simulink model "px4_multirotor_sim"  (R2019a)
settings: Solver=FixedStepAuto  StartTime=0.0  StopTime=sim_time  FixedStep=1/sim_freq  RelTol=1e-3
values from neighbouring files (symbols this model uses):
  C_D = [0.064; 0.067; 0.089].*0    [model_parameters.m]
  d = 0.49    [model_parameters.m]
  m = 4.5    [model_parameters.m]
  pos_e_step = [2;3;-4]    [setup_sim.m]
  r_D = 0.0237    [model_parameters.m]
  tau_T = 0.07    [model_parameters.m]
  virtual_controls_mat = [1 1 1 1; -1/sqrt(2) 1/sqrt(2) 1/sqrt(2) -1/sqrt(2); 1/sqrt(2) -1/sqrt(2) 1/sqrt(2) -1/sqrt(2); 1 1 -1 -1]    [model_parameters.m]
  wind = [0; 0; 0]    [model_parameters.m]
  yaw_step = 0    [setup_sim.m]
undefined symbols (not defined in the file or in its folder): br_filt_denom, br_filt_num, DiscIntNeverNeededParam, eta_w, g, hover_perc, hover_T, K_dp, K_ep, K_np, K_pd, K_phi, K_pi, K_pp, K_psi, K_qd, K_qi, K_qp, K_rd, K_ri, K_rp, K_theta, K_ud, K_ui, K_up, K_vd, K_vi, K_vp, K_wd, K_wi, K_wp, max_T, max_tilt, max_vel_xy, max_vel_z_down, max_vel_z_up, p_int_lim, p_max, q_int_lim, q_max, r_max, rho, thr_max, thr_min, vel_filt_denom, vel_filt_num
libraries: simulink x6, shared6dof x1, sharedtransform x1
settings Model: Creator=anton  LastModifiedBy=anton
settings DataIOCC: ReturnWorkspaceOutputs=off
settings DebuggingCC: ArithmeticOperatorsInVariantConditions=warning
settings ModelReferenceCC: ModelReferenceNumInstancesAllowed=Single

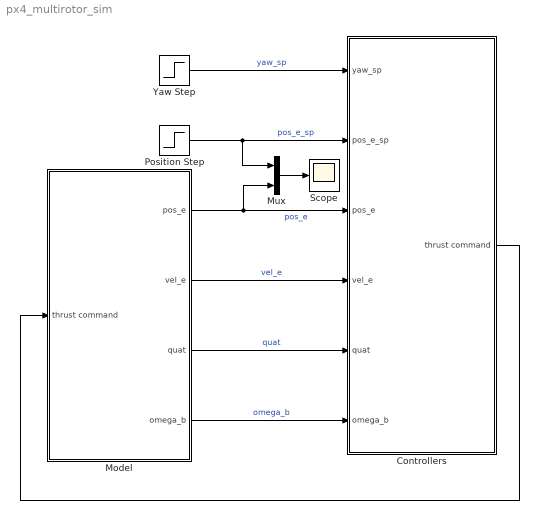
== system px4_multirotor_sim ==
  Controllers : Subsystem
  Model : Subsystem
  Mux : Mux  Inputs=2
  Position Step : Step  Before=[0;0;0]  After=pos_e_step  SampleTime=0
  Scope : Scope
  Yaw Step : Step  After=yaw_step  SampleTime=0
  wires:
  Controllers/1(thrust command) -> Model/1(thrust command)
  Model/1(pos_e) -> Mux/2, Controllers/3(pos_e)  "pos_e"
  Model/2(vel_e) -> Controllers/4(vel_e)  "vel_e"
  Model/3(quat) -> Controllers/5(quat)  "quat"
  Model/4(omega_b) -> Controllers/6(omega_b)  "omega_b"
  Position Step/1 -> Mux/1, Controllers/2(pos_e_sp)  "pos_e_sp"
  Yaw Step/1 -> Controllers/1(yaw_sp)  "yaw_sp"
  Mux/1 -> Scope/1

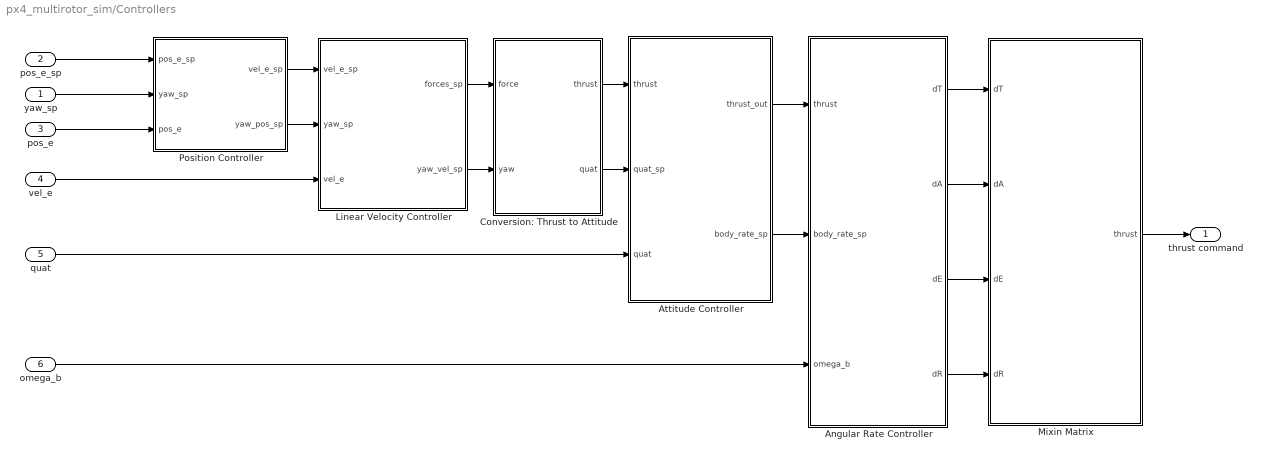
== system px4_multirotor_sim/Controllers ==
  yaw_sp : Inport
  pos_e_sp : Inport  Port=2
  pos_e : Inport  Port=3
  vel_e : Inport  Port=4
  quat : Inport  Port=5
  omega_b : Inport  Port=6
  Angular Rate Controller : Subsystem
  Attitude Controller : Subsystem
  Conversion: Thrust to Attitude : Subsystem
  Linear Velocity Controller : Subsystem
  Mixin Matrix : Subsystem
  Position Controller : Subsystem
  thrust command : Outport
  wires:
  Conversion: Thrust to Attitude/2(quat) -> Attitude Controller/2(quat_sp)
  Mixin Matrix/1(thrust) -> thrust command/1
  vel_e/1 -> Linear Velocity Controller/3(vel_e)
  Angular Rate Controller/3(dE) -> Mixin Matrix/3(dE)
  Attitude Controller/1(thrust_out) -> Angular Rate Controller/1(thrust)
  omega_b/1 -> Angular Rate Controller/3(omega_b)
  yaw_sp/1 -> Position Controller/2(yaw_sp)
  Linear Velocity Controller/2(yaw_vel_sp) -> Conversion: Thrust to Attitude/2(yaw)
  Angular Rate Controller/1(dT) -> Mixin Matrix/1(dT)
  pos_e_sp/1 -> Position Controller/1(pos_e_sp)
  Position Controller/1(vel_e_sp) -> Linear Velocity Controller/1(vel_e_sp)
  quat/1 -> Attitude Controller/3(quat)
  Angular Rate Controller/4(dR) -> Mixin Matrix/4(dR)
  Linear Velocity Controller/1(forces_sp) -> Conversion: Thrust to Attitude/1(force)
  pos_e/1 -> Position Controller/3(pos_e)
  Conversion: Thrust to Attitude/1(thrust) -> Attitude Controller/1(thrust)
  Position Controller/2(yaw_pos_sp) -> Linear Velocity Controller/2(yaw_sp)
  Angular Rate Controller/2(dA) -> Mixin Matrix/2(dA)
  Attitude Controller/2(body_rate_sp) -> Angular Rate Controller/2(body_rate_sp)

== system px4_multirotor_sim/Model ==
  thrust command : Inport
  6 DOF : Subsystem
  Forces and Moments : Subsystem
  Motor Model : Subsystem
  pos_e : Outport
  vel_e : Outport  Port=2
  quat : Outport  Port=3
  omega_b : Outport  Port=4
  wires:
  thrust command/1 -> Motor Model/1(thrust_cmd)
  Forces and Moments/2(moments) -> 6 DOF/2(moments)
  Forces and Moments/1(forces) -> 6 DOF/1(forces)
  6 DOF/1(pos_e) -> pos_e/1, Forces and Moments/1(pos_e)
  6 DOF/2(quat) -> quat/1, Forces and Moments/2(quat)
  6 DOF/3(vel_b) -> Forces and Moments/3(vel_b)
  6 DOF/4(omega_b) -> omega_b/1
  6 DOF/5(vel_e) -> vel_e/1
  Motor Model/1(force) -> Forces and Moments/4(Thrust Commands)

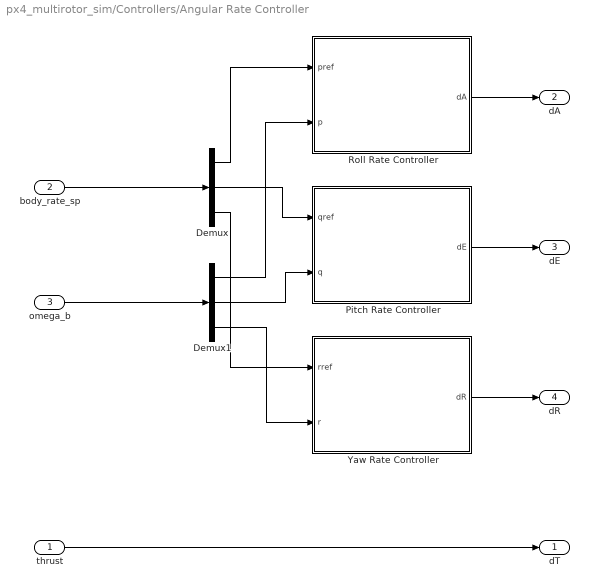
== system px4_multirotor_sim/Controllers/Angular Rate Controller ==
  thrust : Inport
  body_rate_sp : Inport  Port=2
  omega_b : Inport  Port=3
  Demux : Demux  Outputs=3
  Demux1 : Demux  Outputs=3
  Pitch Rate Controller : Subsystem
  Roll Rate Controller : Subsystem
  Yaw Rate Controller : Subsystem
  dT : Outport
  dA : Outport  Port=2
  dE : Outport  Port=3
  dR : Outport  Port=4
  wires:
  Demux1/3 -> Yaw Rate Controller/2(r)
  Demux/3 -> Yaw Rate Controller/1(rref)
  Demux1/1 -> Roll Rate Controller/2(p)
  thrust/1 -> dT/1
  Yaw Rate Controller/1(dR) -> dR/1
  Pitch Rate Controller/1(dE) -> dE/1
  Demux1/2 -> Pitch Rate Controller/2(q)
  Roll Rate Controller/1(dA) -> dA/1
  Demux/1 -> Roll Rate Controller/1(pref)
  Demux/2 -> Pitch Rate Controller/1(qref)
  omega_b/1 -> Demux1/1
  body_rate_sp/1 -> Demux/1

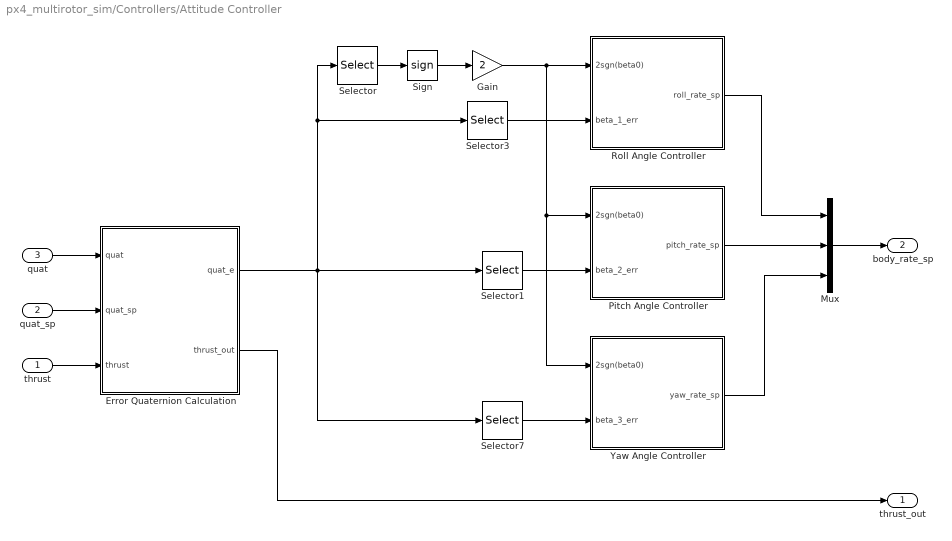
== system px4_multirotor_sim/Controllers/Attitude Controller ==
  thrust : Inport  PortDimensions=1
  quat_sp : Inport  Port=2  PortDimensions=4
  quat : Inport  Port=3  PortDimensions=4
  Error Quaternion Calculation : MATLAB Function  TreatAsAtomicUnit=on
  Gain : Gain  Gain=2
  Mux : Mux  Inputs=3
  Pitch Angle Controller : Subsystem
  Roll Angle Controller : Subsystem
  Selector : Selector  InputPortWidth=4  IndexOptions=Index vector (dialog)  Indices=1  OutputSizes=1
  Selector1 : Selector  InputPortWidth=4  IndexOptions=Index vector (dialog)  Indices=3  OutputSizes=1
  Selector3 : Selector  InputPortWidth=4  IndexOptions=Index vector (dialog)  Indices=2  OutputSizes=1
  Selector7 : Selector  InputPortWidth=4  IndexOptions=Index vector (dialog)  Indices=4  OutputSizes=1
  Sign : Signum
  Yaw Angle Controller : Subsystem
  thrust_out : Outport
  body_rate_sp : Outport  Port=2
  wires:
  Pitch Angle Controller/1(pitch_rate_sp) -> Mux/2
  Selector7/1 -> Yaw Angle Controller/2(beta_3_err)
  Mux/1 -> body_rate_sp/1
  quat/1 -> Error Quaternion Calculation/1(quat)
  quat_sp/1 -> Error Quaternion Calculation/2(quat_sp)
  Error Quaternion Calculation/1(quat_e) -> Selector7/1, Selector/1, Selector3/1, Selector1/1
  Selector/1 -> Sign/1
  Yaw Angle Controller/1(yaw_rate_sp) -> Mux/3
  Roll Angle Controller/1(roll_rate_sp) -> Mux/1
  Selector3/1 -> Roll Angle Controller/2(beta_1_err)
  Gain/1 -> Yaw Angle Controller/1(2sgn(beta0)), Pitch Angle Controller/1(2sgn(beta0)), Roll Angle Controller/1(2sgn(beta0))
  thrust/1 -> Error Quaternion Calculation/3(thrust)
  Sign/1 -> Gain/1
  Error Quaternion Calculation/2(thrust_out) -> thrust_out/1
  Selector1/1 -> Pitch Angle Controller/2(beta_2_err)

== system px4_multirotor_sim/Controllers/Conversion: Thrust to Attitude ==
  force : Inport
  yaw : Inport  Port=2
  thrust2att : MATLAB Function  TreatAsAtomicUnit=on
  thrust : Outport
  quat : Outport  Port=2
  wires:
  yaw/1 -> thrust2att/2(yaw)
  force/1 -> thrust2att/1(force)
  thrust2att/2(thrust) -> thrust/1
  thrust2att/1(quat) -> quat/1

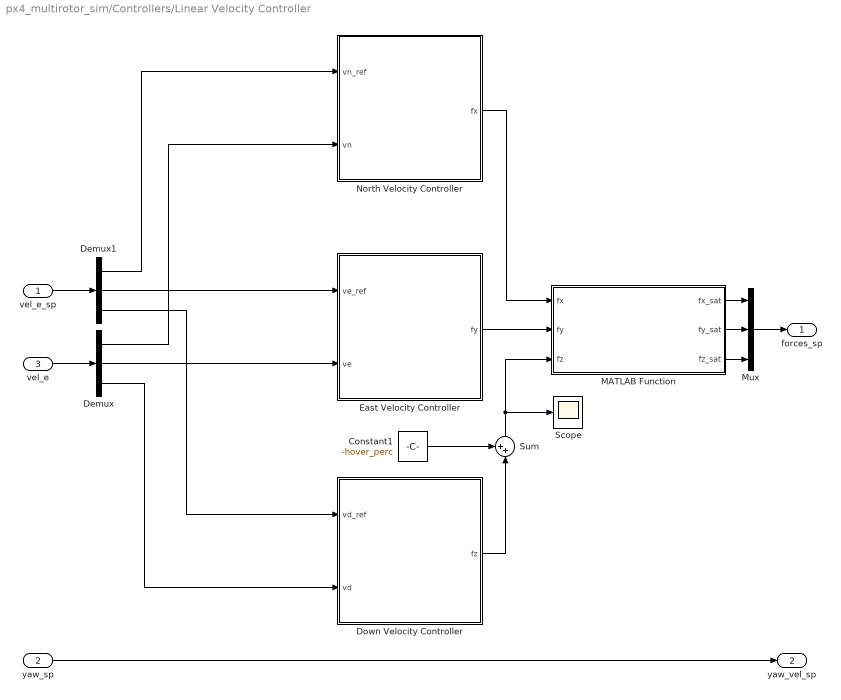
== system px4_multirotor_sim/Controllers/Linear Velocity Controller ==
  vel_e_sp : Inport
  yaw_sp : Inport  Port=2
  vel_e : Inport  Port=3
  Constant1 : Constant  Value=-hover_perc
  Demux : Demux  Outputs=3
  Demux1 : Demux  Outputs=3
  Down Velocity Controller : Subsystem
  East Velocity Controller : Subsystem
  MATLAB Function : MATLAB Function  TreatAsAtomicUnit=on
  Mux : Mux  Inputs=3
  North Velocity Controller : Subsystem
  Scope : Scope
  Sum : Sum  Inputs=++|
  forces_sp : Outport
  yaw_vel_sp : Outport  Port=2
  wires:
  Mux/1 -> forces_sp/1
  Demux/2 -> East Velocity Controller/2(ve)
  vel_e_sp/1 -> Demux1/1
  Down Velocity Controller/1(fz) -> Sum/2
  Demux1/1 -> North Velocity Controller/1(vn_ref)
  Constant1/1 -> Sum/1
  Demux/1 -> North Velocity Controller/2(vn)
  Demux/3 -> Down Velocity Controller/2(vd)
  vel_e/1 -> Demux/1
  MATLAB Function/1(fx_sat) -> Mux/1
  East Velocity Controller/1(fy) -> MATLAB Function/2(fy)
  North Velocity Controller/1(fx) -> MATLAB Function/1(fx)
  yaw_sp/1 -> yaw_vel_sp/1
  Demux1/3 -> Down Velocity Controller/1(vd_ref)
  Demux1/2 -> East Velocity Controller/1(ve_ref)
  MATLAB Function/3(fz_sat) -> Mux/3
  Sum/1 -> Scope/1, MATLAB Function/3(fz)
  MATLAB Function/2(fy_sat) -> Mux/2

== system px4_multirotor_sim/Controllers/Mixin Matrix ==
  dT : Inport
  dA : Inport  Port=2
  dE : Inport  Port=3
  dR : Inport  Port=4
  MATLAB Function : MATLAB Function  TreatAsAtomicUnit=on
  Precision Conversion : Subsystem
  Saturation : Saturate  UpperLimit=1  LowerLimit=0
  thrust : Outport
  wires:
  MATLAB Function/1(thrust) -> Saturation/1
  dT/1 -> MATLAB Function/1(dT)
  Saturation/1 -> Precision Conversion/1(analog_cmd)
  dE/1 -> MATLAB Function/3(dE)
  dA/1 -> MATLAB Function/2(dA)
  dR/1 -> MATLAB Function/4(dR)
  Precision Conversion/1(discrete_cmd) -> thrust/1

== system px4_multirotor_sim/Controllers/Position Controller ==
  pos_e_sp : Inport
  yaw_sp : Inport  Port=2
  pos_e : Inport  Port=3
  Demux : Demux  Outputs=3
  Demux1 : Demux  Outputs=3
  Down Position Controller : Subsystem
  East Position Controller : Subsystem
  Mux : Mux  Inputs=3
  North Position Controller : Subsystem
  vel_e_sp : Outport
  yaw_pos_sp : Outport  Port=2
  wires:
  Demux/1 -> North Position Controller/1(n_ref)
  North Position Controller/1(vn) -> Mux/1
  pos_e_sp/1 -> Demux/1
  yaw_sp/1 -> yaw_pos_sp/1
  Demux1/1 -> North Position Controller/2(n)
  Demux/2 -> East Position Controller/1(e_ref)
  Down Position Controller/1(vd) -> Mux/3
  Demux1/2 -> East Position Controller/2(e)
  Demux/3 -> Down Position Controller/1(d_ref)
  Mux/1 -> vel_e_sp/1
  East Position Controller/1(ve) -> Mux/2
  Demux1/3 -> Down Position Controller/2(d)
  pos_e/1 -> Demux1/1

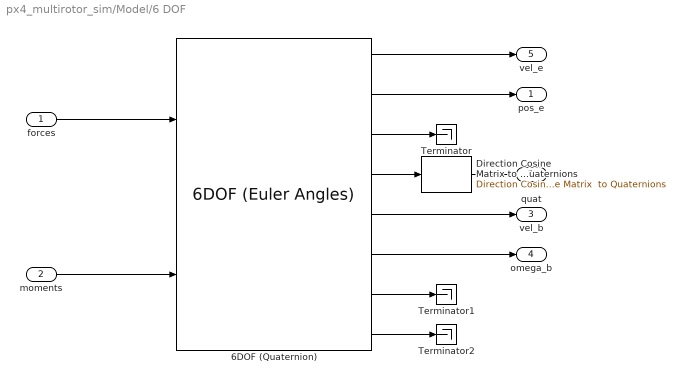
== system px4_multirotor_sim/Model/6 DOF ==
  forces : Inport
  moments : Inport  Port=2
  6DOF (Quaternion) : shared6dof/6DOF (Euler Angles)  units=Metric (MKS)  mtype=Fixed  rep=Quaternion  xme_0=[0 0 0]  Vm_0=[0 0 0]  eul_0=[0 0 0]  pm_0=[0 0 0]  mass_0=m  mass_e=0.5  mass_f=2.0  inertia=I  inertia_e=eye(3)  inertia_f=2*eye(3)  k_quat=2  vre_flag=on  abi_flag=off  aMode=0  xme_statename=''  Vm_statename=''  eul_statename=''  quat_statename=''  pm_statename=''  mass_statename=''
      settings: SourceProductBaseCode=AE
  Direction Cosine Matrix to Quaternions : sharedtransform/Direction Cosine Matrix  to Quaternions  aMode=0  action=None  tolerance=eps(2)
      settings: SourceProductName=Aerospace Blockset  SourceProductBaseCode=AE
  Terminator : Terminator
  Terminator1 : Terminator
  Terminator2 : Terminator
  pos_e : Outport
  quat : Outport  Port=2
  vel_b : Outport  Port=3
  omega_b : Outport  Port=4
  vel_e : Outport  Port=5
  wires:
  6DOF (Quaternion)/4 -> Direction Cosine Matrix to Quaternions/1
  6DOF (Quaternion)/1 -> vel_e/1
  Direction Cosine Matrix to Quaternions/1 -> quat/1
  forces/1 -> 6DOF (Quaternion)/1
  6DOF (Quaternion)/6 -> omega_b/1
  6DOF (Quaternion)/2 -> pos_e/1
  6DOF (Quaternion)/5 -> vel_b/1
  6DOF (Quaternion)/7 -> Terminator1/1
  6DOF (Quaternion)/3 -> Terminator/1
  moments/1 -> 6DOF (Quaternion)/2
  6DOF (Quaternion)/8 -> Terminator2/1

== system px4_multirotor_sim/Model/Forces and Moments ==
  pos_e : Inport
  quat : Inport  Port=2
  vel_b : Inport  Port=3
  Thrust Commands : Inport  Port=4
  Aerodynamic Model : Subsystem
  Gravity Model : Subsystem
  Sum : Sum  Inputs=|+++|
  Sum1 : Sum  Inputs=|+++|
  Thrust Model : Subsystem
  forces : Outport
  moments : Outport  Port=2
  wires:
  Thrust Model/2(moments) -> Sum1/2
  Gravity Model/2(moments) -> Sum1/3
  Gravity Model/1(forces) -> Sum/3
  Aerodynamic Model/2(moments) -> Sum1/1
  Aerodynamic Model/1(forces) -> Sum/1
  Thrust Model/1(forces) -> Sum/2
  Sum/1 -> forces/1
  Sum1/1 -> moments/1
  vel_b/1 -> Aerodynamic Model/1(vel_b)
  pos_e/1 -> Aerodynamic Model/2(pos_e)
  quat/1 -> Gravity Model/1(quat), Aerodynamic Model/3(quat)
  Thrust Commands/1 -> Thrust Model/1(Thrust Commands)

== system px4_multirotor_sim/Model/Motor Model ==
  thrust_cmd : Inport
  Linear Gain : Gain  Gain=max_T
  force : Outport
  wires:
  thrust_cmd/1 -> Linear Gain/1
  Linear Gain/1 -> force/1

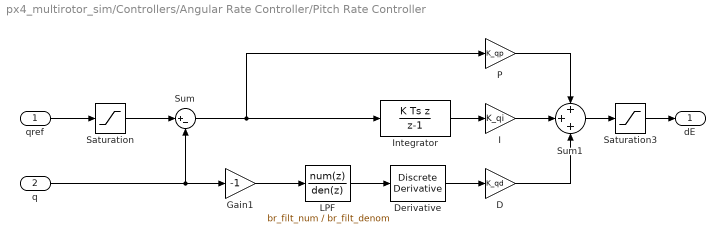
== system px4_multirotor_sim/Controllers/Angular Rate Controller/Pitch Rate Controller ==
  qref : Inport
  q : Inport  Port=2
  D : Gain  Gain=K_qd
  Derivative : simulink/Discrete/Discrete Derivative  gainval=1  ICPrevScaledInput=0.0  OutMin=[]  OutMax=[]  OutDataType=fixdt(1, 16)  OutScaling=2^-10  DoSatur=off
  Gain1 : Gain  Gain=-1
  I : Gain  Gain=K_qi
  Integrator : DiscreteIntegrator  IntegratorMethod=Integration: Backward Euler  gainval=1  SampleTime=-1  LimitOutput=on  UpperSaturationLimit=p_int_lim  LowerSaturationLimit=-p_int_lim  ICPrevOutput=DiscIntNeverNeededParam  ICPrevScaledInput=DiscIntNeverNeededParam
  LPF : DiscreteTransferFcn  Numerator=br_filt_num  Denominator=br_filt_denom
  P : Gain  Gain=K_qp
  Saturation : Saturate  UpperLimit=q_max  LowerLimit=-q_max
  Saturation3 : Saturate  UpperLimit=1  LowerLimit=-1
  Sum : Sum  Inputs=|+-
  Sum1 : Sum  Inputs=+++
  dE : Outport
  wires:
  Gain1/1 -> LPF/1
  P/1 -> Sum1/1
  Sum1/1 -> Saturation3/1
  Saturation/1 -> Sum/1
  I/1 -> Sum1/2
  Sum/1 -> Integrator/1, P/1
  Derivative/1 -> D/1
  D/1 -> Sum1/3
  qref/1 -> Saturation/1
  q/1 -> Gain1/1, Sum/2
  LPF/1 -> Derivative/1
  Integrator/1 -> I/1
  Saturation3/1 -> dE/1

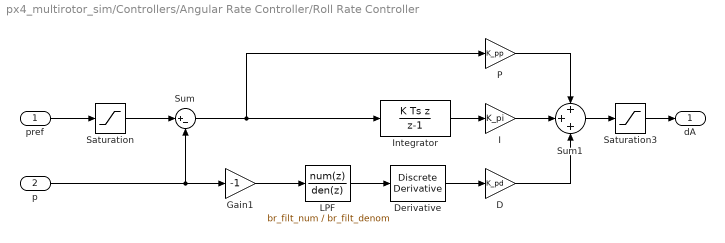
== system px4_multirotor_sim/Controllers/Angular Rate Controller/Roll Rate Controller ==
  pref : Inport
  p : Inport  Port=2
  D : Gain  Gain=K_pd
  Derivative : simulink/Discrete/Discrete Derivative  gainval=1  ICPrevScaledInput=0.0  OutMin=[]  OutMax=[]  OutDataType=fixdt(1, 16)  OutScaling=2^-10  DoSatur=off
  Gain1 : Gain  Gain=-1
  I : Gain  Gain=K_pi
  Integrator : DiscreteIntegrator  IntegratorMethod=Integration: Backward Euler  gainval=1  SampleTime=-1  LimitOutput=on  UpperSaturationLimit=p_int_lim  LowerSaturationLimit=-p_int_lim  ICPrevOutput=DiscIntNeverNeededParam  ICPrevScaledInput=DiscIntNeverNeededParam
  LPF : DiscreteTransferFcn  Numerator=br_filt_num  Denominator=br_filt_denom
  P : Gain  Gain=K_pp
  Saturation : Saturate  UpperLimit=p_max  LowerLimit=-p_max
  Saturation3 : Saturate  UpperLimit=1  LowerLimit=-1
  Sum : Sum  Inputs=|+-
  Sum1 : Sum  Inputs=+++
  dA : Outport
  wires:
  Gain1/1 -> LPF/1
  P/1 -> Sum1/1
  Sum1/1 -> Saturation3/1
  Saturation/1 -> Sum/1
  I/1 -> Sum1/2
  Sum/1 -> Integrator/1, P/1
  Derivative/1 -> D/1
  D/1 -> Sum1/3
  pref/1 -> Saturation/1
  p/1 -> Gain1/1, Sum/2
  LPF/1 -> Derivative/1
  Integrator/1 -> I/1
  Saturation3/1 -> dA/1

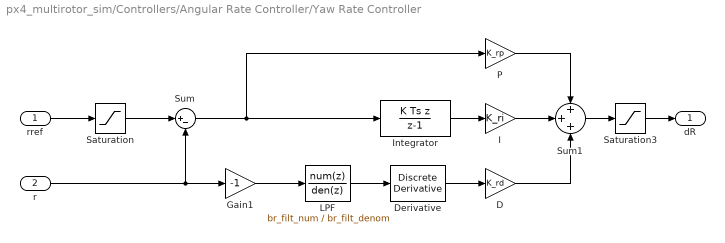
== system px4_multirotor_sim/Controllers/Angular Rate Controller/Yaw Rate Controller ==
  rref : Inport
  r : Inport  Port=2
  D : Gain  Gain=K_rd
  Derivative : simulink/Discrete/Discrete Derivative  gainval=1  ICPrevScaledInput=0.0  OutMin=[]  OutMax=[]  OutDataType=fixdt(1, 16)  OutScaling=2^-10  DoSatur=off
  Gain1 : Gain  Gain=-1
  I : Gain  Gain=K_ri
  Integrator : DiscreteIntegrator  IntegratorMethod=Integration: Backward Euler  gainval=1  SampleTime=-1  LimitOutput=on  UpperSaturationLimit=p_int_lim  LowerSaturationLimit=-p_int_lim  ICPrevOutput=DiscIntNeverNeededParam  ICPrevScaledInput=DiscIntNeverNeededParam
  LPF : DiscreteTransferFcn  Numerator=br_filt_num  Denominator=br_filt_denom
  P : Gain  Gain=K_rp
  Saturation : Saturate  UpperLimit=r_max  LowerLimit=-r_max
  Saturation3 : Saturate  UpperLimit=1  LowerLimit=-1
  Sum : Sum  Inputs=|+-
  Sum1 : Sum  Inputs=+++
  dR : Outport
  wires:
  Gain1/1 -> LPF/1
  P/1 -> Sum1/1
  Sum1/1 -> Saturation3/1
  Saturation/1 -> Sum/1
  I/1 -> Sum1/2
  Sum/1 -> Integrator/1, P/1
  Derivative/1 -> D/1
  D/1 -> Sum1/3
  rref/1 -> Saturation/1
  r/1 -> Gain1/1, Sum/2
  LPF/1 -> Derivative/1
  Integrator/1 -> I/1
  Saturation3/1 -> dR/1

== system px4_multirotor_sim/Controllers/Attitude Controller/Pitch Angle Controller ==
  2sgn(beta0) : Inport
  beta_2_err : Inport  Port=2
  Multiply : Product
  P : Gain  Gain=K_theta
  pitch_rate_sp : Outport
  wires:
  P/1 -> Multiply/1
  beta_2_err/1 -> P/1
  2sgn(beta0)/1 -> Multiply/2
  Multiply/1 -> pitch_rate_sp/1

== system px4_multirotor_sim/Controllers/Attitude Controller/Roll Angle Controller ==
  2sgn(beta0) : Inport
  beta_1_err : Inport  Port=2
  Multiply : Product
  P : Gain  Gain=K_phi
  roll_rate_sp : Outport
  wires:
  P/1 -> Multiply/1
  beta_1_err/1 -> P/1
  2sgn(beta0)/1 -> Multiply/2
  Multiply/1 -> roll_rate_sp/1

== system px4_multirotor_sim/Controllers/Attitude Controller/Yaw Angle Controller ==
  2sgn(beta0) : Inport
  beta_3_err : Inport  Port=2
  Multiply : Product
  P : Gain  Gain=K_psi
  yaw_rate_sp : Outport
  wires:
  P/1 -> Multiply/1
  beta_3_err/1 -> P/1
  2sgn(beta0)/1 -> Multiply/2
  Multiply/1 -> yaw_rate_sp/1

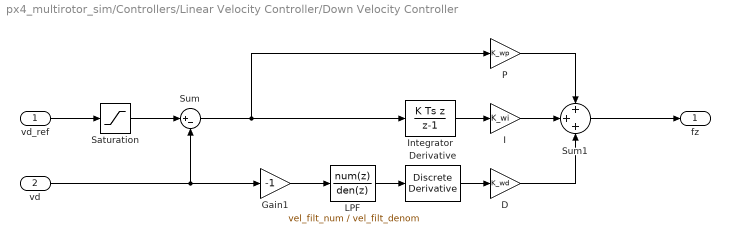
== system px4_multirotor_sim/Controllers/Linear Velocity Controller/Down Velocity Controller ==
  vd_ref : Inport
  vd : Inport  Port=2
  D : Gain  Gain=K_wd
  Derivative : simulink/Discrete/Discrete Derivative  gainval=1  ICPrevScaledInput=0.0  OutMin=[]  OutMax=[]  OutDataType=fixdt(1, 16)  OutScaling=2^-10  DoSatur=off
  Gain1 : Gain  Gain=-1
  I : Gain  Gain=K_wi
  Integrator : DiscreteIntegrator  IntegratorMethod=Integration: Backward Euler  gainval=1  SampleTime=-1  UpperSaturationLimit=q_int_lim  LowerSaturationLimit=-q_int_lim  ICPrevOutput=DiscIntNeverNeededParam  ICPrevScaledInput=DiscIntNeverNeededParam
  LPF : DiscreteTransferFcn  Numerator=vel_filt_num  Denominator=vel_filt_denom
  P : Gain  Gain=K_wp
  Saturation : Saturate  UpperLimit=max_vel_z_up  LowerLimit=max_vel_z_down
  Sum : Sum  Inputs=|+-
  Sum1 : Sum  Inputs=+++
  fz : Outport
  wires:
  vd_ref/1 -> Saturation/1
  P/1 -> Sum1/1
  Sum1/1 -> fz/1
  vd/1 -> Sum/2, Gain1/1
  Gain1/1 -> LPF/1
  LPF/1 -> Derivative/1
  D/1 -> Sum1/3
  Saturation/1 -> Sum/1
  I/1 -> Sum1/2
  Integrator/1 -> I/1
  Sum/1 -> Integrator/1, P/1
  Derivative/1 -> D/1

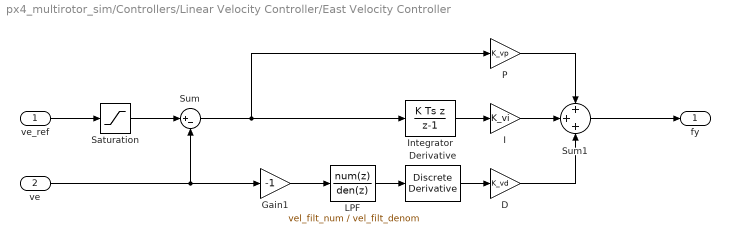
== system px4_multirotor_sim/Controllers/Linear Velocity Controller/East Velocity Controller ==
  ve_ref : Inport
  ve : Inport  Port=2
  D : Gain  Gain=K_vd
  Derivative : simulink/Discrete/Discrete Derivative  gainval=1  ICPrevScaledInput=0.0  OutMin=[]  OutMax=[]  OutDataType=fixdt(1, 16)  OutScaling=2^-10  DoSatur=off
  Gain1 : Gain  Gain=-1
  I : Gain  Gain=K_vi
  Integrator : DiscreteIntegrator  IntegratorMethod=Integration: Backward Euler  gainval=1  SampleTime=-1  UpperSaturationLimit=q_int_lim  LowerSaturationLimit=-q_int_lim  ICPrevOutput=DiscIntNeverNeededParam  ICPrevScaledInput=DiscIntNeverNeededParam
  LPF : DiscreteTransferFcn  Numerator=vel_filt_num  Denominator=vel_filt_denom
  P : Gain  Gain=K_vp
  Saturation : Saturate  UpperLimit=max_vel_xy  LowerLimit=-max_vel_xy
  Sum : Sum  Inputs=|+-
  Sum1 : Sum  Inputs=+++
  fy : Outport
  wires:
  ve_ref/1 -> Saturation/1
  P/1 -> Sum1/1
  Sum1/1 -> fy/1
  ve/1 -> Sum/2, Gain1/1
  Gain1/1 -> LPF/1
  LPF/1 -> Derivative/1
  D/1 -> Sum1/3
  Saturation/1 -> Sum/1
  I/1 -> Sum1/2
  Integrator/1 -> I/1
  Sum/1 -> Integrator/1, P/1
  Derivative/1 -> D/1

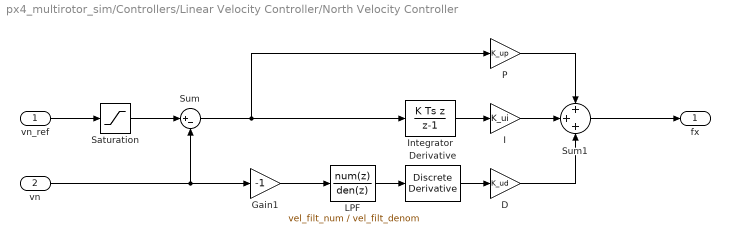
== system px4_multirotor_sim/Controllers/Linear Velocity Controller/North Velocity Controller ==
  vn_ref : Inport
  vn : Inport  Port=2
  D : Gain  Gain=K_ud
  Derivative : simulink/Discrete/Discrete Derivative  gainval=1  ICPrevScaledInput=0.0  OutMin=[]  OutMax=[]  OutDataType=fixdt(1, 16)  OutScaling=2^-10  DoSatur=off
  Gain1 : Gain  Gain=-1
  I : Gain  Gain=K_ui
  Integrator : DiscreteIntegrator  IntegratorMethod=Integration: Backward Euler  gainval=1  SampleTime=-1  UpperSaturationLimit=q_int_lim  LowerSaturationLimit=-q_int_lim  ICPrevOutput=DiscIntNeverNeededParam  ICPrevScaledInput=DiscIntNeverNeededParam
  LPF : DiscreteTransferFcn  Numerator=vel_filt_num  Denominator=vel_filt_denom
  P : Gain  Gain=K_up
  Saturation : Saturate  UpperLimit=max_vel_xy  LowerLimit=-max_vel_xy
  Sum : Sum  Inputs=|+-
  Sum1 : Sum  Inputs=+++
  fx : Outport
  wires:
  vn_ref/1 -> Saturation/1
  P/1 -> Sum1/1
  Sum1/1 -> fx/1
  vn/1 -> Sum/2, Gain1/1
  LPF/1 -> Derivative/1
  D/1 -> Sum1/3
  Saturation/1 -> Sum/1
  I/1 -> Sum1/2
  Integrator/1 -> I/1
  Sum/1 -> Integrator/1, P/1
  Derivative/1 -> D/1
  Gain1/1 -> LPF/1

== system px4_multirotor_sim/Controllers/Mixin Matrix/Precision Conversion ==
  analog_cmd : Inport
  Gain : Gain  Gain=10000
  Gain1 : Gain  Gain=1/10000
  Round : Rounding
  discrete_cmd : Outport
  wires:
  analog_cmd/1 -> Gain/1
  Gain/1 -> Round/1
  Round/1 -> Gain1/1
  Gain1/1 -> discrete_cmd/1

== system px4_multirotor_sim/Controllers/Position Controller/Down Position Controller ==
  d_ref : Inport
  d : Inport  Port=2
  P : Gain  Gain=K_dp
  Sum : Sum  Inputs=|+-
  vd : Outport
  wires:
  d/1 -> Sum/2
  d_ref/1 -> Sum/1
  Sum/1 -> P/1
  P/1 -> vd/1

== system px4_multirotor_sim/Controllers/Position Controller/East Position Controller ==
  e_ref : Inport
  e : Inport  Port=2
  P : Gain  Gain=K_ep
  Sum : Sum  Inputs=|+-
  ve : Outport
  wires:
  e/1 -> Sum/2
  e_ref/1 -> Sum/1
  Sum/1 -> P/1
  P/1 -> ve/1

== system px4_multirotor_sim/Controllers/Position Controller/North Position Controller ==
  n_ref : Inport
  n : Inport  Port=2
  P : Gain  Gain=K_np
  Sum : Sum  Inputs=|+-
  vn : Outport
  wires:
  n/1 -> Sum/2
  n_ref/1 -> Sum/1
  Sum/1 -> P/1
  P/1 -> vn/1

== system px4_multirotor_sim/Model/Forces and Moments/Aerodynamic Model ==
  vel_b : Inport
  pos_e : Inport  Port=2
  quat : Inport  Port=3
  Constant : Constant  Value=wind
  MATLAB Function : MATLAB Function  TreatAsAtomicUnit=on
  forces : Outport
  moments : Outport  Port=2
  wires:
  Constant/1 -> MATLAB Function/2(vw_i)
  MATLAB Function/2(moments) -> moments/1
  quat/1 -> MATLAB Function/4(quat)
  vel_b/1 -> MATLAB Function/1(v_b)
  pos_e/1 -> MATLAB Function/3(ned)
  MATLAB Function/1(forces) -> forces/1

== system px4_multirotor_sim/Model/Forces and Moments/Gravity Model ==
  quat : Inport
  MATLAB Function : MATLAB Function  TreatAsAtomicUnit=on
  forces : Outport
  moments : Outport  Port=2
  wires:
  MATLAB Function/2(moments) -> moments/1
  MATLAB Function/1(forces) -> forces/1
  quat/1 -> MATLAB Function/1(quat)

== system px4_multirotor_sim/Model/Forces and Moments/Thrust Model ==
  Thrust Commands : Inport
  Integrator : Integrator  InitialCondition=hover_T * ones(4,1)
  MATLAB Function : MATLAB Function  TreatAsAtomicUnit=on
  forces : Outport
  moments : Outport  Port=2
  wires:
  MATLAB Function/1(T_dot) -> Integrator/1
  Integrator/1 -> MATLAB Function/1(T)
  Thrust Commands/1 -> MATLAB Function/2(Tc)
  MATLAB Function/2(forces) -> forces/1
  MATLAB Function/3(moments) -> moments/1

== matlab function px4_multirotor_sim/Model/Forces and Moments/Aerodynamic Model/MATLAB Function ==
  data: v_b input size=3; vw_i input size=3; ned input size=3; quat input size=4; rho parameter size=1; forces output size=3; moments output size=3; C_D parameter size=3; eta_w parameter size=1
function [forces, moments] = aerodynamicModel(v_b, vw_i, ned, quat, rho, C_D, eta_w)
    coder.extrinsic("quatrotate");
    
    % Initialize
    vw_b = [0; 0; 0];
    
    vw_b = quatrotate(quat', vw_i')';
    vw_bm = (power(abs(ned(3))/10, eta_w)) .* vw_b;
    v_bw = -v_b + vw_bm;
    q = 0.5 * rho * v_bw.*abs(v_bw);
    
    forces = q.*C_D;
    moments = [0; 0; 0];
    
end

== matlab function px4_multirotor_sim/Model/Forces and Moments/Thrust Model/MATLAB Function ==
  data: T input size=4; T_dot output size=4; Tc input size=4; tau_T parameter size=1; forces output size=3; moments output size=3; d parameter size=1; r_D parameter size=1; virtual_controls_mat parameter size=[4,4]
function [T_dot, forces, moments]  = thrustModel(T, Tc, tau_T, d, r_D, virtual_controls_mat)

    virt_T = virtual_controls_mat * T;

    T_dot = (-T + Tc)/tau_T;
    forces = [0; 0; -virt_T(1)];
    moments = [d*virt_T(2); d*virt_T(3); r_D*virt_T(4)];
    
end

== matlab function px4_multirotor_sim/Model/Forces and Moments/Gravity Model/MATLAB Function ==
  data: quat input size=4; forces output size=3; moments output size=3; m parameter size=1; g parameter size=1
function [forces,moments] = gravitationalModel(quat, m, g)
    coder.extrinsic("quatrotate");

    % Initialize
    forces = [0; 0; 0];
    
    moments = [0 ; 0 ; 0];
    forces = quatrotate(quat', [0 ; 0 ; m*g]')';

end

== matlab function px4_multirotor_sim/Controllers/Linear Velocity Controller/MATLAB Function ==
  data: fx input; fx_sat output; fy input; fz input; fy_sat output; max_tilt parameter; thr_max parameter; fz_sat output; thr_min parameter
function [fx_sat, fy_sat, fz_sat] = constrain_max_tilt(fx, fy, fz, max_tilt, thr_max, thr_min)
    % First constrain fz.
    if fz > -thr_min
        fz_sat = -thr_min;
    elseif fz < -thr_max
        fz_sat = -thr_max;
    else
        fz_sat = fz;
    end
    
    % Constrain fx and fy
    thrust_max_NE_tilt = abs(fz_sat) * tan(max_tilt * pi/180);
    thrust_max_NE = sqrt(thr_max*thr_max - fz_sat*fz_sat);
    thrust_max_NE = min(thrust_max_NE_tilt, thrust_max_NE);
    
    fx_sat = fx;
    fy_sat = fy;
    
    if dot([fx, fy], [fx, fy]) > thrust_max_NE*thrust_max_NE
        mag = norm([fx, fy]);
        fx_sat = fx / mag * thrust_max_NE;
        fy_sat = fy / mag * thrust_max_NE;
    end
end

== matlab function px4_multirotor_sim/Controllers/Conversion: Thrust to Attitude/thrust2att ==
  data: force input size=3; quat output size=4; yaw input size=1; thrust output size=1
function [quat, thrust] = thrust2att(force, yaw)
    coder.extrinsic('dcm2quat');

        % Initialise quat
    quat = [1; 0; 0; 0];
    
    % Thrust is norm of force
    thrust = norm(force);
    
    % Determine body_z rotation (fit body_z onto z axis of force)
    if thrust > 1e-6
        body_z = -force./thrust;
    else
       body_z = [0; 0; 1]; 
    end
    
    % Determine body_x
    yaw_dir = [-sin(yaw); cos(yaw); 0];
    
    if abs(body_z(3)) > 1e-6
        body_x = cross(yaw_dir, body_z);
        
        if body_z(3) < 0
            body_x = -body_x;
        end
        body_x = body_x ./ norm(body_x);
    else
        body_x = [0; 0; 1];
    end
    
    % Determine body_y
    body_y = cross(body_z, body_x);
    body_y = body_y ./ norm(body_y);
    
    % Calculate rotation
    dcm = [body_x body_y body_z];
    quat = dcm2quat(dcm');
    
    % Normalise quaternion
    quat = quat ./ norm(quat);
    
end

== matlab function px4_multirotor_sim/Controllers/Attitude Controller/Error Quaternion Calculation ==
  data: quat input; quat_sp input; quat_e output; thrust input; thrust_out output
function [quat_e, thrust_out] = error_quat(quat, quat_sp, thrust)
    if quat_sp == [0; 0; 0; 0]
       quat_sp = [1; 0; 0; 0];
    end
    
    quat_e = quatmultiply([quat(1) -quat(2) -quat(3) -quat(4)]./norm(quat), quat_sp');
    thrust_out = thrust;
end

== matlab function px4_multirotor_sim/Controllers/Mixin Matrix/MATLAB Function ==
  data: dT input; thrust output; dA input; dE input; dR input; mixin_mat parameter
function thrust = mixin_mat(dT, dA, dE, dR, mixin_mat)

    thrust = mixin_mat * [dT; dA; dE; dR];

end
